simulink library "dip"  (Simulink 8.2)
settings: Solver=ode45  SolverMode=SingleTasking  StartTime=0.0  StopTime=10.0  RelTol=1e-3
undefined symbols (not defined in the file or in its folder): ENUM_LANELAMPMODE_GREEN, ENUM_LANELAMPMODE_GREY, ENUM_LANELAMPMODE_OFF, ENUM_LANELAMPMODE_RED, ENUM_LFCHMISTATUS_ACTING, ENUM_LFCHMISTATUS_OFF, ENUM_LFCHMISTATUS_STANDBY, ENUM_LFCSTATE_ADASFAILURE, ENUM_LFCSTATE_AUTOSTEERING, ENUM_LFCSTATE_DEGRADED, ENUM_LFCSTATE_DISABLED, ENUM_LFCSTATE_EPSRECOVERYPENDING, ENUM_LFCSTATE_OFF, ENUM_LFCSTATE_SOFTEN, ENUM_LFCSTATE_STANDBY, ENUM_LKAHMISTATUS_ACTING, ENUM_LKAHMISTATUS_OFF, ENUM_LKASTATE_ADASFAILURE, ENUM_LKASTATE_DISABLED, ENUM_LKASTATE_EPSRECOVERYPENDING, ENUM_LKASTATE_LEFTASSISTING, ENUM_LKASTATE_OFF, ENUM_LKASTATE_OPERATIONAL, ENUM_LKASTATE_RIGHTASSISTING, ENUM_LKASTATE_STANDBY, FALSE, KDIP_ADASOnSoundReqLatch_s
libraries: hcu_lib x4, simulink x2
settings Model: Creator=13192  LastModifiedBy=13192

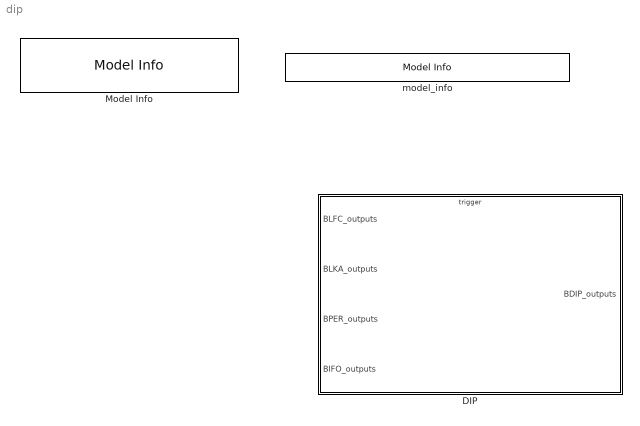
== system dip ==
  DIP : Subsystem
      settings: RTWSystemCode=Nonreusable function  RTWFcnNameOpts=Use subsystem name  RTWFileNameOpts=Use subsystem name
  Model Info : simulink/Model-Wide Utilities/Model Info  InitialBlockCM=None  BlockCM=None  Frame=on  DisplayStringWithTags=|  HorizontalTextAlignment=Left  LeftAlignmentValue=0.02  SourceBlockDiagram=dip  TagMaxNumber=20
      | Model Version        : %<ModelVersion>
      | Creator                   : %<Creator>
      | Last Modified by    : %<LastModifiedBy>
  model_info : simulink/Model-Wide Utilities/Model Info  InitialBlockCM=None  BlockCM=None  Frame=on  DisplayStringWithTags=$Id: hcu_lib.mdl 289 2016-04-11 06:01:08Z chimotsai $  HorizontalTextAlignment=Center  LeftAlignmentValue=0.5  SourceBlockDiagram=dip  TagMaxNumber=20

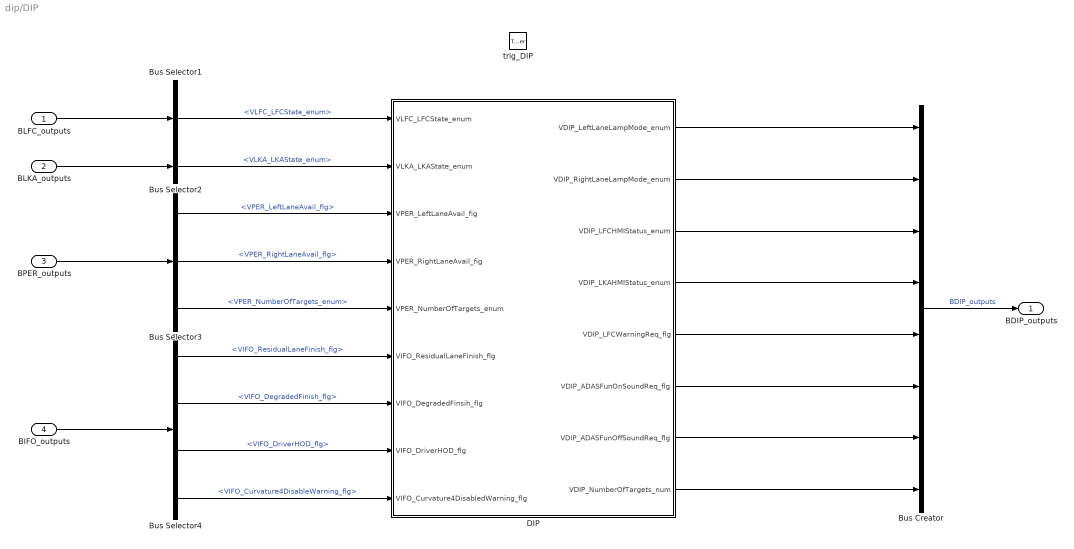
== system dip/DIP ==
  BLFC_outputs : Inport  OutDataTypeStr=Bus: BLFC_outputs
  BLKA_outputs : Inport  Port=2  OutDataTypeStr=Bus: BLKA_outputs
  BPER_outputs : Inport  Port=3  OutDataTypeStr=Bus: BPER_outputs
  BIFO_outputs : Inport  Port=4  OutDataTypeStr=Bus: BIFO_outputs
  trig_DIP : TriggerPort  TriggerType=function-call
  Bus Creator : BusCreator  Inputs=8  OutDataTypeStr=Bus: BDIP_outputs
  Bus Selector1 : BusSelector  OutputSignals=VLFC_LFCState_enum
  Bus Selector2 : BusSelector  OutputSignals=VLKA_LKAState_enum
  Bus Selector3 : BusSelector  OutputSignals=VPER_LeftLaneAvail_flg,VPER_RightLaneAvail_flg,VPER_NumberOfTargets_enum
  Bus Selector4 : BusSelector  OutputSignals=VIFO_ResidualLaneFinish_flg,VIFO_DegradedFinish_flg,VIFO_DriverHOD_flg,VIFO_Curvature4DisableWarning_flg
  DIP : Subsystem
  BDIP_outputs : Outport  OutDataTypeStr=Bus: BDIP_outputs
  wires:
  BLFC_outputs/1 -> Bus Selector1/1
  Bus Creator/1 -> BDIP_outputs/1  "BDIP_outputs"
  Bus Selector1/1 -> DIP/1(VLFC_LFCState_enum)  "<VLFC_LFCState_enum>"
  BLKA_outputs/1 -> Bus Selector2/1
  Bus Selector2/1 -> DIP/2(VLKA_LKAState_enum)  "<VLKA_LKAState_enum>"
  BPER_outputs/1 -> Bus Selector3/1
  Bus Selector3/1 -> DIP/3(VPER_LeftLaneAvail_fig)  "<VPER_LeftLaneAvail_flg>"
  Bus Selector3/2 -> DIP/4(VPER_RightLaneAvail_fig)  "<VPER_RightLaneAvail_flg>"
  DIP/1(VDIP_LeftLaneLampMode_enum) -> Bus Creator/1
  DIP/2(VDIP_RightLaneLampMode_enum) -> Bus Creator/2
  DIP/3(VDIP_LFCHMIStatus_enum) -> Bus Creator/3
  DIP/4(VDIP_LKAHMIStatus_enum) -> Bus Creator/4
  DIP/5(VDIP_LFCWarningReq_flg) -> Bus Creator/5
  DIP/6(VDIP_ADASFunOnSoundReq_flg) -> Bus Creator/6
  DIP/7(VDIP_ADASFunOffSoundReq_flg) -> Bus Creator/7
  Bus Selector3/3 -> DIP/5(VPER_NumberOfTargets_enum)  "<VPER_NumberOfTargets_enum>"
  DIP/8(VDIP_NumberOfTargets_num) -> Bus Creator/8
  BIFO_outputs/1 -> Bus Selector4/1
  Bus Selector4/3 -> DIP/8(VIFO_DriverHOD_flg)  "<VIFO_DriverHOD_flg>"
  Bus Selector4/2 -> DIP/7(VIFO_DegradedFinsih_flg)  "<VIFO_DegradedFinish_flg>"
  Bus Selector4/1 -> DIP/6(VIFO_ResidualLaneFinish_flg)  "<VIFO_ResidualLaneFinish_flg>"
  Bus Selector4/4 -> DIP/9(VIFO_Curvature4DisabledWarning_flg)  "<VIFO_Curvature4DisableWarning_flg>"

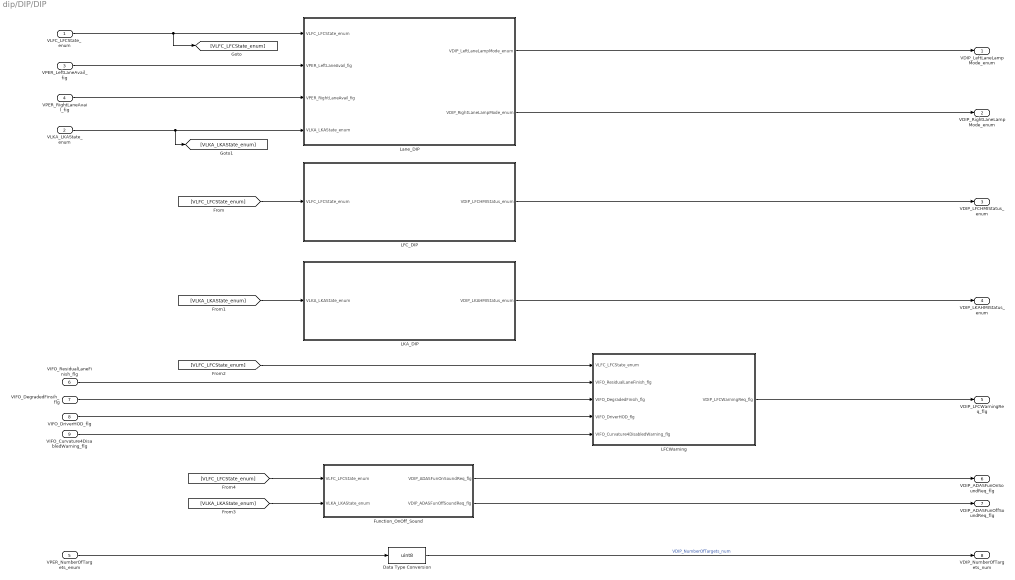
== system dip/DIP/DIP ==
  VLFC_LFCState_enum : Inport
  VLKA_LKAState_enum : Inport  Port=2
  VPER_LeftLaneAvail_fig : Inport  Port=3
  VPER_RightLaneAvail_fig : Inport  Port=4
  VPER_NumberOfTargets_enum : Inport  Port=5
  VIFO_ResidualLaneFinish_flg : Inport  Port=6
  VIFO_DegradedFinsih_flg : Inport  Port=7
  VIFO_DriverHOD_flg : Inport  Port=8
  VIFO_Curvature4DisabledWarning_flg : Inport  Port=9
  Data Type Conversion : DataTypeConversion  OutDataTypeStr=uint8
  Function_OnOff_Sound : Subsystem
  LFCWarning : Subsystem
  LFC_DIP : Stateflow chart  TreatAsAtomicUnit=on
  LKA_DIP : Stateflow chart  TreatAsAtomicUnit=on
  Lane_DIP : Stateflow chart  TreatAsAtomicUnit=on
  VDIP_LeftLaneLampMode_enum : Outport
  VDIP_RightLaneLampMode_enum : Outport  Port=2
  VDIP_LFCHMIStatus_enum : Outport  Port=3
  VDIP_LKAHMIStatus_enum : Outport  Port=4
  VDIP_LFCWarningReq_flg : Outport  Port=5
  VDIP_ADASFunOnSoundReq_flg : Outport  Port=6
  VDIP_ADASFunOffSoundReq_flg : Outport  Port=7
  VDIP_NumberOfTargets_num : Outport  Port=8
  wires:
  VPER_LeftLaneAvail_fig/1 -> Lane_DIP/2(VPER_LeftLaneAvail_fig)
  VPER_RightLaneAvail_fig/1 -> Lane_DIP/3(VPER_RightLaneAvail_fig)
  VLKA_LKAState_enum/1 -> [VLKA_LKAState_enum], Lane_DIP/4(VLKA_LKAState_enum)
  Lane_DIP/1(VDIP_LeftLaneLampMode_enum) -> VDIP_LeftLaneLampMode_enum/1
  Lane_DIP/2(VDIP_RightLaneLampMode_enum) -> VDIP_RightLaneLampMode_enum/1
  LFC_DIP/1(VDIP_LFCHMIStatus_enum) -> VDIP_LFCHMIStatus_enum/1
  LKA_DIP/1(VDIP_LKAHMIStatus_enum) -> VDIP_LKAHMIStatus_enum/1
  Function_OnOff_Sound/1(VDIP_ADASFunOnSoundReq_flg) -> VDIP_ADASFunOnSoundReq_flg/1
  Function_OnOff_Sound/2(VDIP_ADASFunOffSoundReq_flg) -> VDIP_ADASFunOffSoundReq_flg/1
  VPER_NumberOfTargets_enum/1 -> Data Type Conversion/1
  Data Type Conversion/1 -> VDIP_NumberOfTargets_num/1  "VDIP_NumberOfTargets_num"
  VLFC_LFCState_enum/1 -> [VLFC_LFCState_enum], Lane_DIP/1(VLFC_LFCState_enum)
  VIFO_ResidualLaneFinish_flg/1 -> LFCWarning/2(VIFO_ResidualLaneFinish_flg)
  LFCWarning/1(VDIP_LFCWarningReq_flg) -> VDIP_LFCWarningReq_flg/1
  VIFO_DegradedFinsih_flg/1 -> LFCWarning/3(VIFO_DegradedFinsih_flg)
  VIFO_DriverHOD_flg/1 -> LFCWarning/4(VIFO_DriverHOD_flg)
  VIFO_Curvature4DisabledWarning_flg/1 -> LFCWarning/5(VIFO_Curvature4DisabledWarning_flg)
  [VLFC_LFCState_enum] -> LFC_DIP/1(VLFC_LFCState_enum)
  [VLKA_LKAState_enum] -> LKA_DIP/1(VLKA_LKAState_enum)
  [VLFC_LFCState_enum] -> LFCWarning/1(VLFC_LFCState_enum)
  [VLFC_LFCState_enum] -> Function_OnOff_Sound/1(VLFC_LFCState_enum)
  [VLKA_LKAState_enum] -> Function_OnOff_Sound/2(VLKA_LKAState_enum)

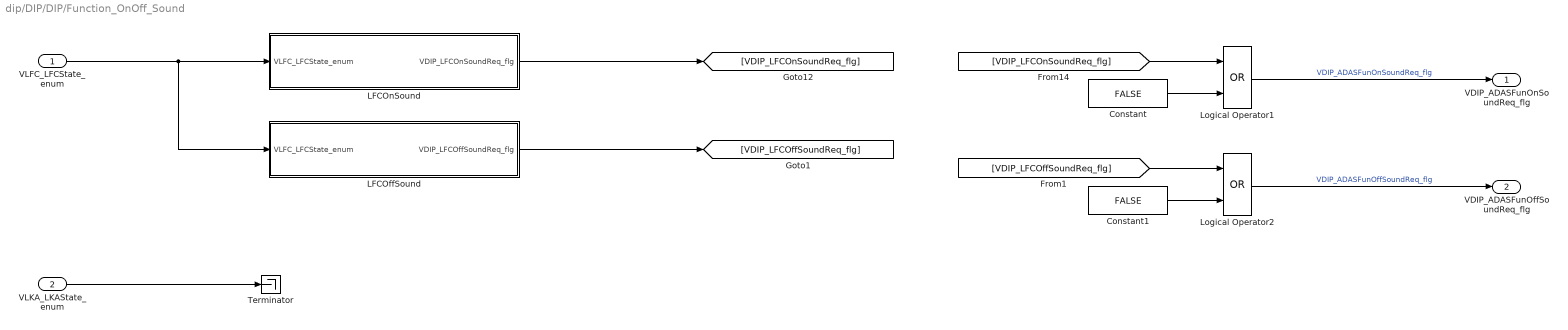
== system dip/DIP/DIP/Function_OnOff_Sound ==
  VLFC_LFCState_enum : Inport
  VLKA_LKAState_enum : Inport  Port=2
  Constant : Constant  Value=FALSE
  Constant1 : Constant  Value=FALSE
  LFCOffSound : Subsystem
  LFCOnSound : Subsystem
  Logical Operator1 : Logic  Operator=OR  AllPortsSameDT=off  OutDataTypeStr=boolean
  Logical Operator2 : Logic  Operator=OR  AllPortsSameDT=off  OutDataTypeStr=boolean
  Terminator : Terminator
  VDIP_ADASFunOnSoundReq_flg : Outport
  VDIP_ADASFunOffSoundReq_flg : Outport  Port=2
  wires:
  VLFC_LFCState_enum/1 -> LFCOffSound/1(VLFC_LFCState_enum), LFCOnSound/1(VLFC_LFCState_enum)
  LFCOnSound/1(VDIP_LFCOnSoundReq_flg) -> [VDIP_LFCOnSoundReq_flg]
  LFCOffSound/1(VDIP_LFCOffSoundReq_flg) -> [VDIP_LFCOffSoundReq_flg]
  [VDIP_LFCOnSoundReq_flg] -> Logical Operator1/1
  Logical Operator1/1 -> VDIP_ADASFunOnSoundReq_flg/1  "VDIP_ADASFunOnSoundReq_flg"
  Logical Operator2/1 -> VDIP_ADASFunOffSoundReq_flg/1  "VDIP_ADASFunOffSoundReq_flg"
  [VDIP_LFCOffSoundReq_flg] -> Logical Operator2/1
  VLKA_LKAState_enum/1 -> Terminator/1
  Constant/1 -> Logical Operator1/2
  Constant1/1 -> Logical Operator2/2

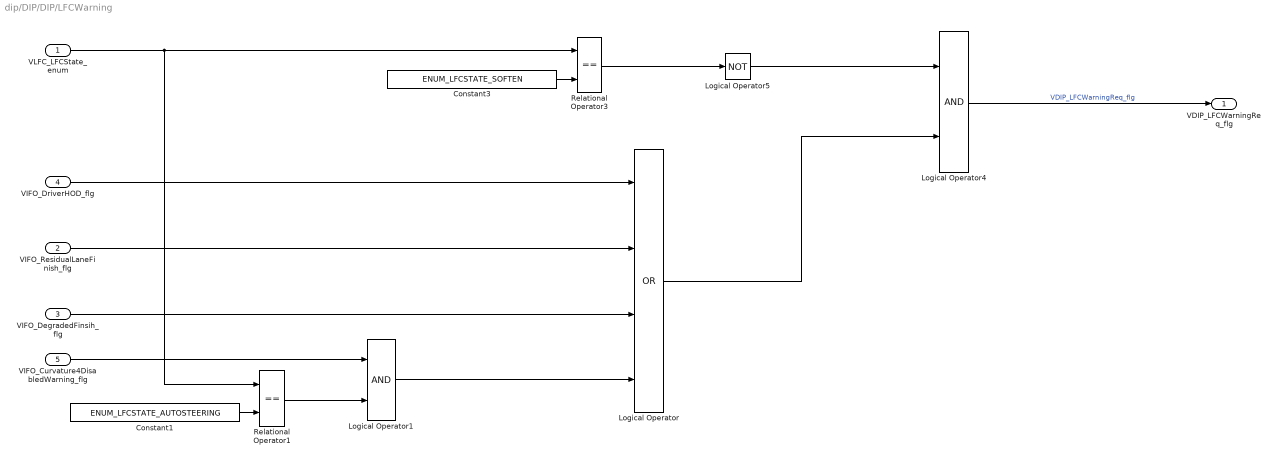
== system dip/DIP/DIP/LFCWarning ==
  VLFC_LFCState_enum : Inport
  VIFO_ResidualLaneFinish_flg : Inport  Port=2
  VIFO_DegradedFinsih_flg : Inport  Port=3
  VIFO_DriverHOD_flg : Inport  Port=4
  VIFO_Curvature4DisabledWarning_flg : Inport  Port=5
  Constant1 : Constant  Value=ENUM_LFCSTATE_AUTOSTEERING
  Constant3 : Constant  Value=ENUM_LFCSTATE_SOFTEN
  Logical Operator : Logic  Operator=OR  Inputs=4  AllPortsSameDT=off  OutDataTypeStr=boolean
  Logical Operator1 : Logic  AllPortsSameDT=off  OutDataTypeStr=boolean
  Logical Operator4 : Logic  AllPortsSameDT=off  OutDataTypeStr=boolean
  Logical Operator5 : Logic  Operator=NOT  AllPortsSameDT=off  OutDataTypeStr=boolean
  Relational Operator1 : RelationalOperator  Operator===  OutDataTypeStr=boolean
  Relational Operator3 : RelationalOperator  Operator===  OutDataTypeStr=boolean
  VDIP_LFCWarningReq_flg : Outport
  wires:
  Logical Operator5/1 -> Logical Operator4/1
  VLFC_LFCState_enum/1 -> Relational Operator1/1, Relational Operator3/1
  Relational Operator3/1 -> Logical Operator5/1
  Constant3/1 -> Relational Operator3/2
  Logical Operator4/1 -> VDIP_LFCWarningReq_flg/1  "VDIP_LFCWarningReq_flg"
  VIFO_DriverHOD_flg/1 -> Logical Operator/1
  VIFO_ResidualLaneFinish_flg/1 -> Logical Operator/2
  VIFO_DegradedFinsih_flg/1 -> Logical Operator/3
  Logical Operator/1 -> Logical Operator4/2
  VIFO_Curvature4DisabledWarning_flg/1 -> Logical Operator1/1
  Constant1/1 -> Relational Operator1/2
  Relational Operator1/1 -> Logical Operator1/2
  Logical Operator1/1 -> Logical Operator/4

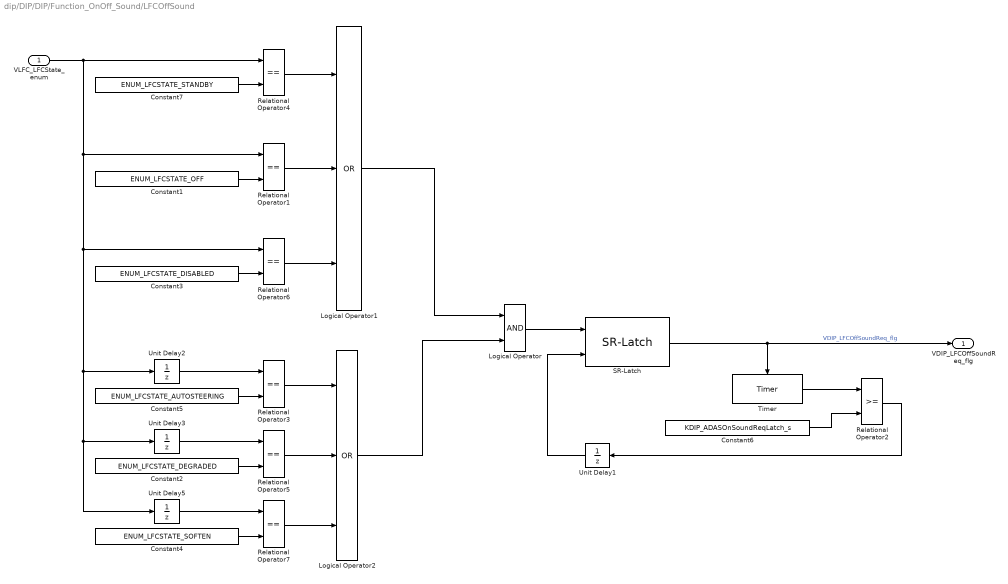
== system dip/DIP/DIP/Function_OnOff_Sound/LFCOffSound ==
  VLFC_LFCState_enum : Inport
  Constant1 : Constant  Value=ENUM_LFCSTATE_OFF
  Constant2 : Constant  Value=ENUM_LFCSTATE_DEGRADED
  Constant3 : Constant  Value=ENUM_LFCSTATE_DISABLED
  Constant4 : Constant  Value=ENUM_LFCSTATE_SOFTEN
  Constant5 : Constant  Value=ENUM_LFCSTATE_AUTOSTEERING
  Constant6 : Constant  Value=KDIP_ADASOnSoundReqLatch_s
  Constant7 : Constant  Value=ENUM_LFCSTATE_STANDBY
  Logical Operator : Logic  AllPortsSameDT=off  OutDataTypeStr=boolean
  Logical Operator1 : Logic  Operator=OR  Inputs=3  AllPortsSameDT=off  OutDataTypeStr=boolean
  Logical Operator2 : Logic  Operator=OR  Inputs=3  AllPortsSameDT=off  OutDataTypeStr=boolean
  Relational Operator{1,3..7} (6 alike) : RelationalOperator  Operator===  OutDataTypeStr=boolean
  Relational Operator2 : RelationalOperator  OutDataTypeStr=boolean
  SR-Latch : hcu_lib/SR-Latch  SystemSampleTime=-1
  Timer : hcu_lib/Timer  SystemSampleTime=-1
  Unit Delay{1..3,5} (4 alike) : UnitDelay  SampleTime=-1
  VDIP_LFCOffSoundReq_flg : Outport
  wires:
  Relational Operator4/1 -> Logical Operator1/1
  Constant5/1 -> Relational Operator3/2
  Logical Operator2/1 -> Logical Operator/2
  Unit Delay1/1 -> SR-Latch/2
  Relational Operator3/1 -> Logical Operator2/1
  Unit Delay5/1 -> Relational Operator7/1
  SR-Latch/1 -> VDIP_LFCOffSoundReq_flg/1, Timer/Enable  "VDIP_LFCOffSoundReq_flg"
  Relational Operator5/1 -> Logical Operator2/2
  Constant4/1 -> Relational Operator7/2
  Relational Operator7/1 -> Logical Operator2/3
  Timer/1 -> Relational Operator2/1
  Unit Delay2/1 -> Relational Operator3/1
  Unit Delay3/1 -> Relational Operator5/1
  Constant2/1 -> Relational Operator5/2
  Constant6/1 -> Relational Operator2/2
  Constant7/1 -> Relational Operator4/2
  Logical Operator/1 -> SR-Latch/1
  Relational Operator2/1 -> Unit Delay1/1
  Constant1/1 -> Relational Operator1/2
  Relational Operator1/1 -> Logical Operator1/2
  Logical Operator1/1 -> Logical Operator/1
  VLFC_LFCState_enum/1 -> Relational Operator4/1, Relational Operator1/1, Relational Operator6/1, Unit Delay5/1, Unit Delay3/1, Unit Delay2/1
  Constant3/1 -> Relational Operator6/2
  Relational Operator6/1 -> Logical Operator1/3

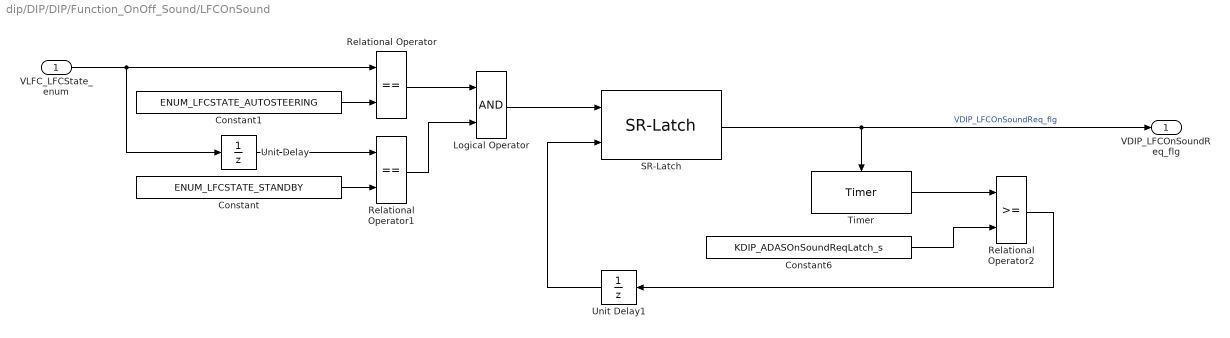
== system dip/DIP/DIP/Function_OnOff_Sound/LFCOnSound ==
  VLFC_LFCState_enum : Inport
  Constant : Constant  Value=ENUM_LFCSTATE_STANDBY
  Constant1 : Constant  Value=ENUM_LFCSTATE_AUTOSTEERING
  Constant6 : Constant  Value=KDIP_ADASOnSoundReqLatch_s
  Logical Operator : Logic  AllPortsSameDT=off  OutDataTypeStr=boolean
  Relational Operator : RelationalOperator  Operator===  OutDataTypeStr=boolean
  Relational Operator1 : RelationalOperator  Operator===  OutDataTypeStr=boolean
  Relational Operator2 : RelationalOperator  OutDataTypeStr=boolean
  SR-Latch : hcu_lib/SR-Latch  SystemSampleTime=-1
  Timer : hcu_lib/Timer  SystemSampleTime=-1
  Unit Delay : UnitDelay  SampleTime=-1
  Unit Delay1 : UnitDelay  SampleTime=-1
  VDIP_LFCOnSoundReq_flg : Outport
  wires:
  Unit Delay/1 -> Relational Operator1/1
  SR-Latch/1 -> VDIP_LFCOnSoundReq_flg/1, Timer/Enable  "VDIP_LFCOnSoundReq_flg"
  Constant1/1 -> Relational Operator/2
  Constant/1 -> Relational Operator1/2
  Constant6/1 -> Relational Operator2/2
  Timer/1 -> Relational Operator2/1
  VLFC_LFCState_enum/1 -> Unit Delay/1, Relational Operator/1
  Unit Delay1/1 -> SR-Latch/2
  Relational Operator2/1 -> Unit Delay1/1
  Relational Operator/1 -> Logical Operator/1
  Relational Operator1/1 -> Logical Operator/2
  Logical Operator/1 -> SR-Latch/1

== stateflow chart DIP/DIP/LFC_DIP ==
  (default) -> (junction 18)
  (junction 18) -> (junction 19) [order 1] : [VLFC_LFCState_enum==ENUM_LFCSTATE_DISABLED || VLFC_LFCState_enum==ENUM_LFCSTATE_OFF || VLFC_LFCState_enum==ENUM_LFCSTATE_ADASFAILURE || VLFC_LFCState_enum==ENUM_LFCSTATE_EPSRECOVERYPENDING]
  (junction 18) -> (junction 20) [order 2]
  (junction 19) -> (junction 27) : {VDIP_LFCHMIStatus_enum=ENUM_LFCHMISTATUS_OFF;}
  (junction 20) -> (junction 21) [order 1] : [VLFC_LFCState_enum==ENUM_LFCSTATE_STANDBY]
  (junction 20) -> (junction 22) [order 2]
  (junction 21) -> (junction 26) : {VDIP_LFCHMIStatus_enum=ENUM_LFCHMISTATUS_STANDBY;}
  (junction 22) -> (junction 23) [order 1] : [VLFC_LFCState_enum==ENUM_LFCSTATE_AUTOSTEERING || VLFC_LFCState_enum==ENUM_LFCSTATE_DEGRADED || VLFC_LFCState_enum==ENUM_LFCSTATE_SOFTEN]
  (junction 22) -> (junction 24) [order 2] : {VDIP_LFCHMIStatus_enum=ENUM_LFCHMISTATUS_OFF;}
  (junction 23) -> (junction 25) : {VDIP_LFCHMIStatus_enum=ENUM_LFCHMISTATUS_ACTING;}
  (junction 25) -> (junction 24)
  (junction 26) -> (junction 25)
  (junction 27) -> (junction 26)
  (junction 31) -> (junction 30)
  (junction 32) -> (junction 31)
  data: VLFC_LFCState_enum input double; VDIP_LFCHMIStatus_enum output double; ENUM_LFCSTATE_DISABLED parameter double; ENUM_LFCSTATE_OFF parameter double; ENUM_LFCSTATE_STANDBY parameter double; ENUM_LFCSTATE_AUTOSTEERING parameter double; ENUM_LFCSTATE_DEGRADED parameter double; ENUM_LFCSTATE_SOFTEN parameter double; ENUM_LFCSTATE_ADASFAILURE parameter double; ENUM_LFCSTATE_EPSRECOVERYPENDING parameter double; ENUM_LFCHMISTATUS_ACTING parameter double; ENUM_LFCHMISTATUS_OFF parameter double; ENUM_LFCHMISTATUS_STANDBY parameter double

== stateflow chart DIP/DIP/LKA_DIP ==
  (default) -> (junction 62)
  (junction 62) -> (junction 63) [order 1] : [VLKA_LKAState_enum==ENUM_LKASTATE_DISABLED || VLKA_LKAState_enum==ENUM_LKASTATE_OFF || VLKA_LKAState_enum==ENUM_LKASTATE_ADASFAILURE ||...
      |  VLKA_LKAState_enum==ENUM_LKASTATE_EPSRECOVERYPENDING || VLKA_LKAState_enum==ENUM_LKASTATE_STANDBY]
  (junction 62) -> (junction 64) [order 2]
  (junction 63) -> (junction 68) : {VDIP_LKAHMIStatus_enum=ENUM_LKAHMISTATUS_OFF;}
  (junction 64) -> (junction 65) [order 1] : [VLKA_LKAState_enum==ENUM_LKASTATE_OPERATIONAL ||...
      |  VLKA_LKAState_enum==ENUM_LKASTATE_LEFTASSISTING || VLKA_LKAState_enum==ENUM_LKASTATE_RIGHTASSISTING]
  (junction 64) -> (junction 66) [order 2] : {VDIP_LKAHMIStatus_enum=ENUM_LKAHMISTATUS_OFF;}
  (junction 65) -> (junction 67) : {VDIP_LKAHMIStatus_enum=ENUM_LKAHMISTATUS_ACTING;}
  (junction 67) -> (junction 66)
  (junction 68) -> (junction 67)
  data: VLKA_LKAState_enum input double; ENUM_LKASTATE_DISABLED parameter double; ENUM_LKASTATE_OFF parameter double; ENUM_LKASTATE_STANDBY parameter double; ENUM_LKASTATE_OPERATIONAL parameter double; ENUM_LKASTATE_LEFTASSISTING parameter double; ENUM_LKASTATE_ADASFAILURE parameter double; ENUM_LKASTATE_EPSRECOVERYPENDING parameter double; VDIP_LKAHMIStatus_enum output double; ENUM_LKAHMISTATUS_OFF parameter double; ENUM_LKAHMISTATUS_ACTING parameter double; ENUM_LKASTATE_RIGHTASSISTING parameter double

== stateflow chart DIP/DIP/Lane_DIP ==
  (default) -> (junction 95)
  (junction 95) -> (junction 96) [order 1] : [VLFC_LFCState_enum==ENUM_LFCSTATE_AUTOSTEERING || VLFC_LFCState_enum==ENUM_LFCSTATE_SOFTEN]
  (junction 95) -> (junction 99) [order 2]
  (junction 96) -> (junction 97)
  (junction 97) -> (junction 98) [order 1] : [VPER_LeftLaneAvail_fig && VPER_RightLaneAvail_fig]
  (junction 97) -> (junction 101) [order 2]
  (junction 98) -> (junction 125) : {VDIP_LeftLaneLampMode_enum=ENUM_LANELAMPMODE_GREEN; ...
      | VDIP_RightLaneLampMode_enum=ENUM_LANELAMPMODE_GREEN;}
  (junction 99) -> (junction 100) [order 1] : [VLFC_LFCState_enum==ENUM_LFCSTATE_DEGRADED]
  (junction 99) -> (junction 105) [order 2]
  (junction 100) -> (junction 121) : {VDIP_LeftLaneLampMode_enum=ENUM_LANELAMPMODE_OFF; ...
      | VDIP_RightLaneLampMode_enum=ENUM_LANELAMPMODE_OFF;}
  (junction 101) -> (junction 102) [order 1] : [VPER_LeftLaneAvail_fig && !VPER_RightLaneAvail_fig]
  (junction 101) -> (junction 103) [order 2]
  (junction 102) -> (junction 124) : {VDIP_LeftLaneLampMode_enum=ENUM_LANELAMPMODE_GREEN; ...
      | VDIP_RightLaneLampMode_enum=ENUM_LANELAMPMODE_OFF;}
  (junction 103) -> (junction 104) [order 1] : [!VPER_LeftLaneAvail_fig && VPER_RightLaneAvail_fig]
  (junction 103) -> (junction 122) [order 2] : {VDIP_LeftLaneLampMode_enum=ENUM_LANELAMPMODE_OFF; ...
      | VDIP_RightLaneLampMode_enum=ENUM_LANELAMPMODE_OFF;}
  (junction 104) -> (junction 123) : {VDIP_LeftLaneLampMode_enum=ENUM_LANELAMPMODE_OFF; ...
      | VDIP_RightLaneLampMode_enum=ENUM_LANELAMPMODE_GREEN;}
  (junction 105) -> (junction 106) [order 1] : [VLKA_LKAState_enum==ENUM_LKASTATE_LEFTASSISTING]
  (junction 105) -> (junction 107) [order 2]
  (junction 106) -> (junction 120) : {VDIP_LeftLaneLampMode_enum=ENUM_LANELAMPMODE_RED;}
  (junction 107) -> (junction 108) [order 1] : [VLKA_LKAState_enum==ENUM_LKASTATE_RIGHTASSISTING]
  (junction 107) -> (junction 109) [order 2]
  (junction 108) -> (junction 119) : {VDIP_RightLaneLampMode_enum=ENUM_LANELAMPMODE_RED;}
  (junction 109) -> (junction 110) [order 1] : [VPER_LeftLaneAvail_fig && VPER_RightLaneAvail_fig]
  (junction 109) -> (junction 111) [order 2]
  (junction 110) -> (junction 118) : {VDIP_LeftLaneLampMode_enum=ENUM_LANELAMPMODE_GREY; ...
      | VDIP_RightLaneLampMode_enum=ENUM_LANELAMPMODE_GREY;}
  (junction 111) -> (junction 112) [order 1] : [VPER_LeftLaneAvail_fig && !VPER_RightLaneAvail_fig]
  (junction 111) -> (junction 113) [order 2]
  (junction 112) -> (junction 117) : {VDIP_LeftLaneLampMode_enum=ENUM_LANELAMPMODE_GREY; ...
      | VDIP_RightLaneLampMode_enum=ENUM_LANELAMPMODE_OFF;}
  (junction 113) -> (junction 114) [order 1] : [!VPER_LeftLaneAvail_fig && VPER_RightLaneAvail_fig]
  (junction 113) -> (junction 115) [order 2] : {VDIP_LeftLaneLampMode_enum=ENUM_LANELAMPMODE_OFF; ...
      | VDIP_RightLaneLampMode_enum=ENUM_LANELAMPMODE_OFF;}
  (junction 114) -> (junction 116) : {VDIP_LeftLaneLampMode_enum=ENUM_LANELAMPMODE_OFF; ...
      | VDIP_RightLaneLampMode_enum=ENUM_LANELAMPMODE_GREY;}
  (junction 116) -> (junction 115)
  (junction 117) -> (junction 116)
  (junction 118) -> (junction 117)
  (junction 119) -> (junction 118)
  (junction 120) -> (junction 119)
  (junction 121) -> (junction 120)
  (junction 122) -> (junction 121)
  (junction 123) -> (junction 122)
  (junction 124) -> (junction 123)
  (junction 125) -> (junction 124)
  (junction 126) -> (junction 125)
  (junction 127) -> (junction 126)
  (junction 128) -> (junction 127)
  data: VLFC_LFCState_enum input double; ENUM_LFCSTATE_AUTOSTEERING parameter double; ENUM_LFCSTATE_DEGRADED parameter double; ENUM_LANELAMPMODE_GREEN parameter double; ENUM_LANELAMPMODE_OFF parameter double; VDIP_LeftLaneLampMode_enum output double; VDIP_RightLaneLampMode_enum output double; VPER_LeftLaneAvail_fig input double; VPER_RightLaneAvail_fig input double; ENUM_LANELAMPMODE_RED parameter double; ENUM_LANELAMPMODE_GREY parameter double; ENUM_LFCSTATE_SOFTEN parameter double; VLKA_LKAState_enum input double; ENUM_LKASTATE_LEFTASSISTING parameter double; ENUM_LKASTATE_RIGHTASSISTING parameter double
